simulink model "Model_Control_Cascaded"  (R2021a)
settings: Solver=VariableStepAuto  StartTime=0.0  StopTime=100  RelTol=1e-3
values from neighbouring files (symbols this model uses):
  Ts = 1/fs    (= 0.05)    [Identification.m]    (also in Model_Verification.m)
undefined symbols (not defined in the file or in its folder): sigbuilder_block
settings Model: Creator=moesaab  LastModifiedBy=moesaab

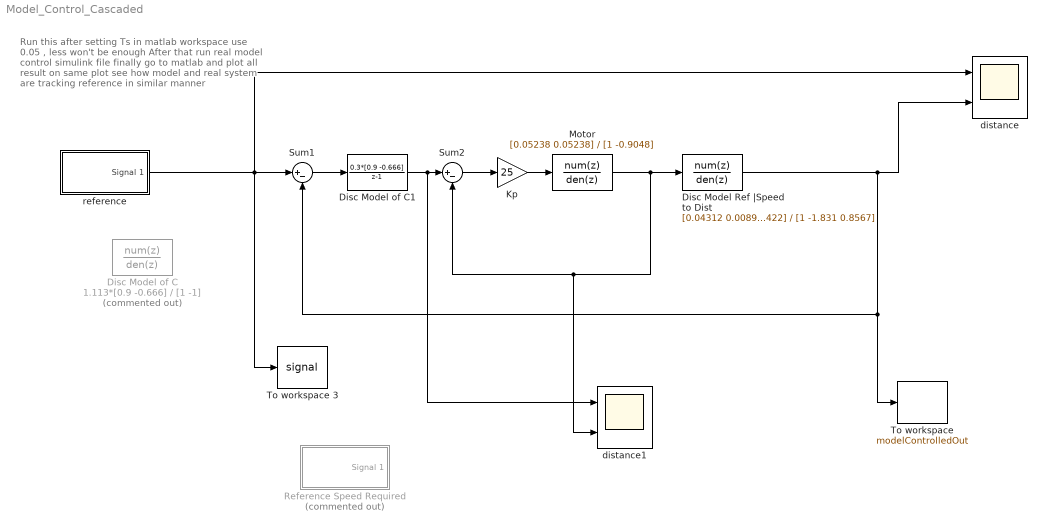
== system Model_Control_Cascaded ==
  note: Run this after setting Ts in matlab workspace
      |  use 0.05 , less won't be enough
      | After that run real model control simulink file
      | finally go to matlab and plot all result on same plot
      | see how model and real system are tracking
      | reference in similar manner
  Disc Model Ref |Speed to Dist : DiscreteTransferFcn  Numerator=[0.04312 0.008904 -0.03422]  Denominator=[1 -1.831 0.8567]  SampleTime=Ts
  Disc Model of C : DiscreteTransferFcn  Commented=on  Numerator=1.113*[0.9 -0.666]  Denominator=[1 -1]  SampleTime=Ts
  Disc Model of C1 : DiscreteTransferFcn  Numerator=0.3*[0.9 -0.666]  Denominator=[1 -1]  SampleTime=0.05
  Kp : Gain  Gain=25
  Motor : DiscreteTransferFcn  Numerator=[0.05238 0.05238]  Denominator=[1 -0.9048]  SampleTime=Ts
  Reference Speed Required : Subsystem  Tag=STV Subsys  Commented=on  LoadFcn=sigbuilder_block('load');  StartFcn=sigbuilder_block('start');  StopFcn=sigbuilder_block('stop');  ClipboardFcn=sigbuilder_block('clipboard');  mask(Sigbuilder block){tuvar=[0:10]}
      mask help: Simulink:masks:SigbuilderBlock_MD
      mask init:
      | if ~strcmp(get_param(bdroot(gcbh),'SimulationStatus'),'stopped') tuvar = sigbuilder_block('maskInit'); end
      settings: CopyFcn=sigbuilder_block('copy');  DeleteFcn=sigbuilder_block('delete');  ModelCloseFcn=sigbuilder_block('modelClose');  PreSaveFcn=sigbuilder_block('preSave');  PauseFcn=sigbuilder_block('pause');  ContinueFcn=sigbuilder_block('continue');  NameChangeFcn=sigbuilder_block('namechange');  OpenFcn=sigbuilder_block('open',[66.297 56.3168 1228.99 491.168 ]);  CloseFcn=sigbuilder_block('close');
      mask Display: plot(0, 0, 100, 100,[2, 2, 32, 32, 2], [68, 8, 8, 68, 68],[32, 2], [38, 38], [32, 19, 2],[53, 60, 44], [32, 17, 17, 2],[16, 16, 31, 31]);txt = getActiveGroup(gcbh);text(2, 100, txt,'verticalAlignment', 'top');
  Sum1 : Sum  Inputs=|+-
  Sum2 : Sum  Inputs=|+-
  To workspace : ToWorkspace  VariableName=modelControlledOut  SampleTime=Ts
      settings: Save2DSignal=2-D array (concatenate along first dimension)
  To workspace 3 : ToWorkspace  VariableName=signal  SampleTime=Ts
      settings: Save2DSignal=2-D array (concatenate along first dimension)
  distance : Scope  NumInputPorts=2
  distance1 : Scope  NumInputPorts=2
  "reference " : Subsystem  Tag=STV Subsys  LoadFcn=sigbuilder_block('load');  StartFcn=sigbuilder_block('start');  StopFcn=sigbuilder_block('stop');  ClipboardFcn=sigbuilder_block('clipboard');  mask(Sigbuilder block){tuvar=[0:10]}
      mask help: Simulink:masks:SigbuilderBlock_MD
      mask init:
      | if ~strcmp(get_param(bdroot(gcbh),'SimulationStatus'),'stopped') tuvar = sigbuilder_block('maskInit'); end
      settings: CopyFcn=sigbuilder_block('copy');  DeleteFcn=sigbuilder_block('delete');  ModelCloseFcn=sigbuilder_block('modelClose');  PreSaveFcn=sigbuilder_block('preSave');  PauseFcn=sigbuilder_block('pause');  ContinueFcn=sigbuilder_block('continue');  NameChangeFcn=sigbuilder_block('namechange');  OpenFcn=sigbuilder_block('open',[49.901 0 666.535 680.079 ]);  CloseFcn=sigbuilder_block('close');
      mask Display: plot(0, 0, 100, 100,[2, 2, 32, 32, 2], [68, 8, 8, 68, 68],[32, 2], [38, 38], [32, 19, 2],[53, 60, 44], [32, 17, 17, 2],[16, 16, 31, 31]);txt = getActiveGroup(gcbh);text(2, 100, txt,'verticalAlignment', 'top');
  wires:
  Disc Model Ref |Speed to Dist/1 -> Sum1/2, To workspace/1, distance/2
  "reference "/1(Signal 1) -> distance/1, To workspace 3/1, Sum1/1
  Kp/1 -> Motor/1
  Sum2/1 -> Kp/1
  Motor/1 -> distance1/2, Sum2/2, Disc Model Ref |Speed to Dist/1
  Disc Model of C1/1 -> distance1/1, Sum2/1
  Sum1/1 -> Disc Model of C1/1

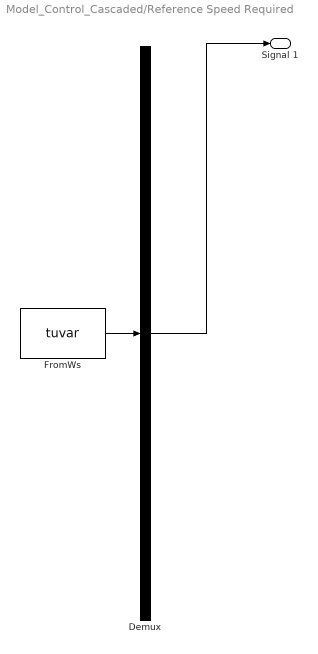
== system Model_Control_Cascaded/Reference Speed Required ==
  Demux : Demux  Tag=STV Demux  Outputs=1
      settings: DisplayOption=none
  FromWs : FromWorkspace  Tag=STV FromWs  VariableName=tuvar  SampleTime=Ts
      SigBuilderData=|
      | common.afterFinalStr = 'Extrapolate'
      | common.sampleTime = 'Ts'
      | dataSet.timeRange = [0 50]
      | dataSet.name = 'Group 1'
      | sbobj.Groups.Name = 'Group 1'
      | sbobj.Groups.Signals.Name = 'Signal 1'
      | sbobj.Groups.Signals.XData = [0 6.3 6.3 10.1 10.1 15.25 15.25 18.05 18.05 22.1 22.1 29.8 29.8 35.1 35.1 39.7 39.7 50]
      | sbobj.Groups.Signals.YData = [0.698 0.698 0.899 0.899 1.001 1.001 0.798 0.798 0.721 0.721 0.898359090909 0.898534090909 1.129 1.129 1.002 1.002 0.942 0.942]
      | sbobj.Groups.TimeRange = [0 50]
  Signal 1 : Outport  Tag=STV Outport
  wires:
  Demux/1 -> Signal 1/1
  FromWs/1 -> Demux/1

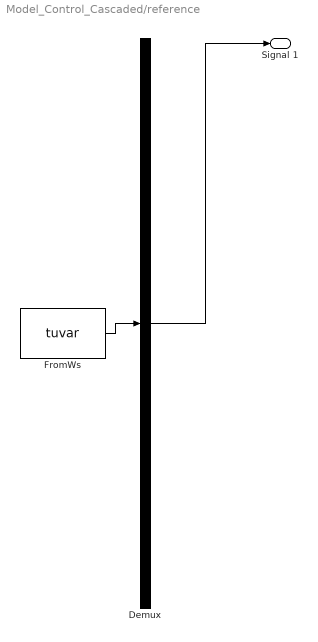
== system Model_Control_Cascaded/reference  ==
  Demux : Demux  Tag=STV Demux  Outputs=1
      settings: DisplayOption=none
  FromWs : FromWorkspace  Tag=STV FromWs  VariableName=tuvar  SampleTime=0.05  ZeroCross=off  OutputAfterFinalValue=Setting to zero
      SigBuilderData=|
      | common.afterFinalStr = 'Set to zero'
      | common.sampleTime = '0.05'
      | dataSet.timeRange = [0 100]
      | dataSet.name = 'Group 1'
      | sbobj.Groups.Name = 'Group 1'
      | sbobj.Groups.Signals.Name = 'Signal 1'
      | sbobj.Groups.Signals.XData = [0 10.6 10.6 24.4 24.4 36 36 45.9 45.9 59.7 59.7 81.7 81.7 100]
      | sbobj.Groups.Signals.YData = [1.7 1.7 1.915 1.915 2.024 2.024 1.858 1.858 2.112 2.112 1.772 1.772 2.328 2.328]
      | sbobj.Groups.TimeRange = [0 100]
  Signal 1 : Outport  Tag=STV Outport
  wires:
  Demux/1 -> Signal 1/1
  FromWs/1 -> Demux/1
